simulink model "LADRC4"  (R2023a)
settings: Solver=VariableStepAuto  StartTime=0.0  StopTime=10.0  RelTol=1e-3
settings Model: Creator=belov  LastModifiedBy=belov

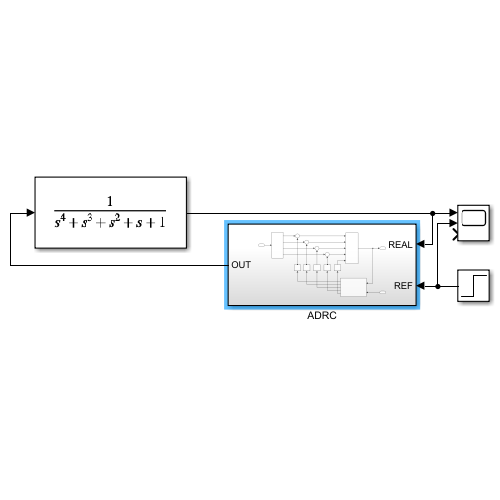
[thumbnail: Simulink's stored preview of the top-level diagram]
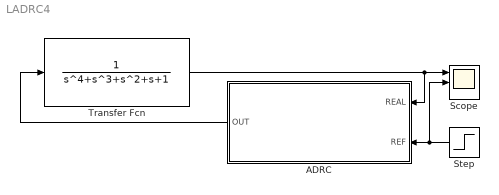
== system LADRC4 ==
  ADRC : Subsystem
  Scope : Scope  NumInputPorts=3
  Step : Step  SampleTime=0
  Transfer Fcn : TransferFcn  Denominator=[1 1 1 1 1]
  wires:
  Step/1 -> ADRC/2(REF), Scope/2
  Transfer Fcn/1 -> ADRC/1(REAL), Scope/1
  ADRC/1(OUT) -> Transfer Fcn/1

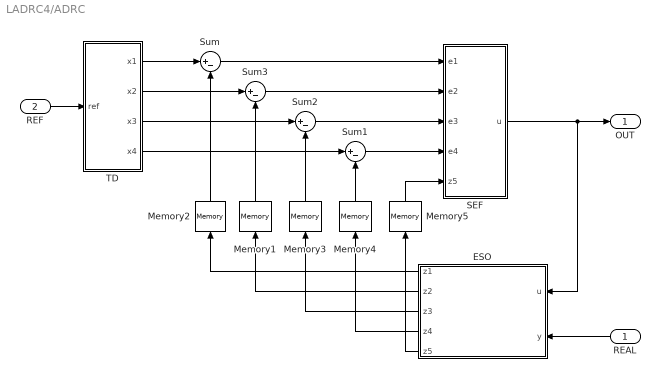
== system LADRC4/ADRC ==
  REAL : Inport
  REF : Inport  Port=2
  ESO : MATLAB Function  TreatAsAtomicUnit=on  SystemSampleTime=0.001
  Memory{1..5} (5 alike) : Memory
  SEF : MATLAB Function  TreatAsAtomicUnit=on  SystemSampleTime=0.001
  Sum{,1..3} (4 alike) : Sum  Inputs=|+-
  TD : MATLAB Function  TreatAsAtomicUnit=on  SystemSampleTime=0.001
  OUT : Outport
  wires:
  REF/1 -> TD/1(ref)
  Memory3/1 -> Sum2/2
  Memory1/1 -> Sum3/2
  Memory2/1 -> Sum/2
  ESO/4(z4) -> Memory4/1
  ESO/3(z3) -> Memory3/1
  ESO/2(z2) -> Memory1/1
  ESO/1(z1) -> Memory2/1
  Sum2/1 -> SEF/3(e3)
  Sum3/1 -> SEF/2(e2)
  TD/3(x3) -> Sum2/1
  TD/2(x2) -> Sum3/1
  Sum/1 -> SEF/1(e1)
  TD/1(x1) -> Sum/1
  REAL/1 -> ESO/2(y)
  TD/4(x4) -> Sum1/1
  Memory4/1 -> Sum1/2
  Sum1/1 -> SEF/4(e4)
  ESO/5(z5) -> Memory5/1
  Memory5/1 -> SEF/5(z5)
  SEF/1(u) -> ESO/1(u), OUT/1

== matlab function LADRC4/ADRC/SEF ==
  data: e1 input; u output; e2 input; e3 input; e4 input; z5 input
function u = SEF(e1, e2, e3, e4, z5)

b0 = 1;

wc = 7;

a1 = wc * wc * wc * wc;
a2 = 4 * wc * wc * wc;
a3 = 6 * wc * wc;
a4 = 4 * wc;
u0 = a1 * e1 + a2 * e2 + a3 * e3 + a4 * e4;
u = (u0 - z5) / b0;
% u = 1 / b0 * (a1 * e1 + a2 * e2 + a3 * e3 + z4);

end

== matlab function LADRC4/ADRC/TD ==
  data: ref input; x1 output; x2 output; x3 output; x4 output
function [x1, x2, x3, x4] = TD(ref)

persistent x1_ x2_ x3_ x4_;

h = 0.001; % 步长
r = 7;

if isempty(x1_)
    x1_=0;
end
if isempty(x2_)
    x2_=0;
end
if isempty(x3_)
    x3_=0;
end
if isempty(x4_)
    x4_=0;
end

x1 = x1_ + h * x2_;
x2 = x2_ + h * x3_;
x3 = x3_ + h * x4_;
x4 = x4_ - h * (4 * r * x4_ + 6 * r * r * x3_ + 4 * r * r * r * x2_ + r * r * r * r * x1_ - r * r * r * r * ref);

x1_ = x1;
x2_ = x2;
x3_ = x3;
x4_ = x4;

end

== matlab function LADRC4/ADRC/ESO ==
  data: u input; z1 output; y input; z2 output; z3 output; z4 output; z5 output
function [z1, z2, z3, z4, z5] = ESO(u, y)

wo = 35;
b0 = 1;

beta1 = 5 * wo;
beta2 = 10 * wo * wo;
beta3 = 10 * wo * wo * wo;
beta4 = 5 * wo * wo * wo * wo;
beta5 = wo * wo * wo * wo * wo;

h = 0.001;

persistent z1_ z2_ z3_ z4_ z5_;

if isempty(z1_)
    z1_ = 0;
end
if isempty(z2_)
    z2_ = 0;
end
if isempty(z3_)
    z3_ = 0;
end
if isempty(z4_)
    z4_ = 0;
end
if isempty(z5_)
    z5_ = 0;
end

z1 = z1_ + h * (-beta1 * z1_ + z2_ + beta1 * y);
z2 = z2_ + h * (-beta2 * z1_ + z3_ + beta2 * y);
z3 = z3_ + h * (-beta3 * z1_ + z4_ + beta3 * y);
z4 = z4_ + h * (-beta4 * z1_ + z5_ + b0 *  u + beta4 * y);
z5 = z5_ + h * (-beta5 * z1_ + beta5 * y);

z1_ = z1;
z2_ = z2;
z3_ = z3;
z4_ = z4;
z5_ = z5;
end
